simulink model "slip_angle"  (R2015a)
settings: Solver=ode45  StartTime=0.0  StopTime=10.0  RelTol=1e-3
settings Model: Creator=BML  LastModifiedBy=BML

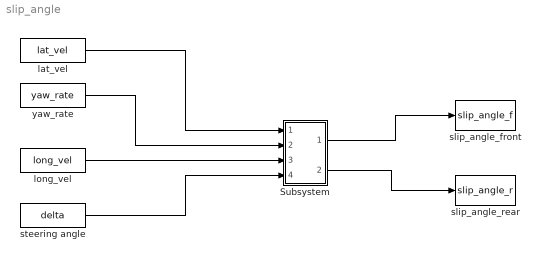
== system slip_angle ==
  Subsystem : Subsystem
  lat_vel : FromWorkspace  VariableName=lat_vel  SampleTime=0
  long_vel : FromWorkspace  VariableName=long_vel  SampleTime=0
  slip_angle_front : ToWorkspace  VariableName=slip_angle_f  SaveFormat=Timeseries  SampleTime=-1
  slip_angle_rear : ToWorkspace  VariableName=slip_angle_r  SaveFormat=Timeseries  SampleTime=-1
  steering angle : FromWorkspace  VariableName=delta  SampleTime=0
  yaw_rate : FromWorkspace  VariableName=yaw_rate  SampleTime=0
  wires:
  lat_vel/1 -> Subsystem/1(In1)
  yaw_rate/1 -> Subsystem/2(In2)
  long_vel/1 -> Subsystem/3(In3)
  steering angle/1 -> Subsystem/4(In4)
  Subsystem/1(Out1) -> slip_angle_front/1
  Subsystem/2(Out2) -> slip_angle_rear/1

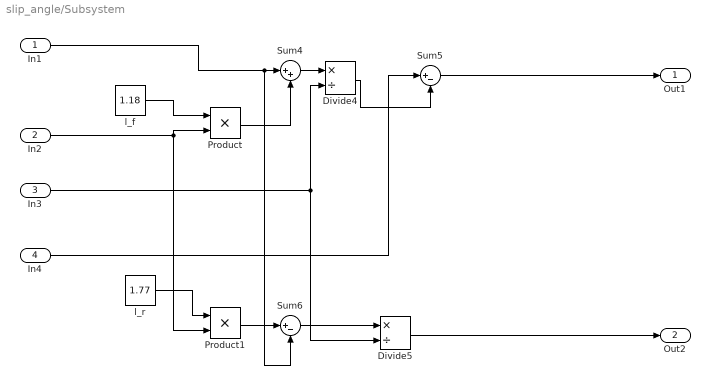
== system slip_angle/Subsystem ==
  In1 : Inport
  In2 : Inport  Port=2
  In3 : Inport  Port=3
  In4 : Inport  Port=4
  Divide4 : Product  Inputs=*/
  Divide5 : Product  Inputs=*/
  Product : Product
  Product1 : Product
  Sum4 : Sum  Inputs=|++
  Sum5 : Sum  Inputs=|+-
  Sum6 : Sum  Inputs=|+-
  l_f : Constant  Value=1.18
  l_r : Constant  Value=1.77
  Out1 : Outport
  Out2 : Outport  Port=2
  wires:
  In2/1 -> Product1/2, Product/2
  In3/1 -> Divide5/2, Divide4/2
  l_f/1 -> Product/1
  In1/1 -> Sum6/2, Sum4/1
  Divide4/1 -> Sum5/2
  Product/1 -> Sum4/2
  Sum4/1 -> Divide4/1
  Divide5/1 -> Out2/1
  In4/1 -> Sum5/1
  Sum5/1 -> Out1/1
  Product1/1 -> Sum6/1
  l_r/1 -> Product1/1
  Sum6/1 -> Divide5/1
